simulink model "Lab_Practice_7_1simulink"  (R2024b)
settings: Solver=ode45  StartTime=0.0  StopTime=t_sim  MaxStep=0.01*Ts  MinStep=0.001*Ts  RelTol=1e-3
values from neighbouring files (symbols this model uses):
  C = [1 0]    [Es1_l7.m]    (also in Lab_Practice_7_1.m; Lab_Practice_7_1.mat; MPC_example_10_12.m = [600 0]; MPC_ratevariation.m = [600 0])
  md = MPCInit(Ad,Bd,Cy,Cz,Dz,Cc,Dc,Hp,Hw,z_blk,Hu,u_blk,du_max,du_min,u_max,u_min,z_max,z_min,Q,R,[],[],h,cmode,'qp_as')    [Es1_l7.m]    (also in Lab_Practice_7_1.m = MPCInit(Ad,Bd,Cy,Cz,Dz,Cc,Dc,Hp,Hw, z_blk, Hc, u_blk, du_max; Lab_Practice_7_1.mat = ; MPC_example_10_12.m; MPC_ratevariation.m)
  Ts = 0.05    [Es1_l7.m]    (also in Lab_Practice_7_1.m; Lab_Practice_7_1.mat; MPC_example_10_12.m = 0.001; MPC_ratevariation.m = 0.001)
  x0 = [1; 0]    [Es1_l7.m]    (also in Lab_Practice_7_1.m = [1;0]; Lab_Practice_7_1.mat = [1 0]; MPC_example_10_12.m = [0;0]; MPC_ratevariation.m = [-0.25;0])
libraries: cstblocks x1
settings Model: Creator=filoz  LastModifiedBy=filoz
settings SolverCC: InitialStep=0.001*Ts

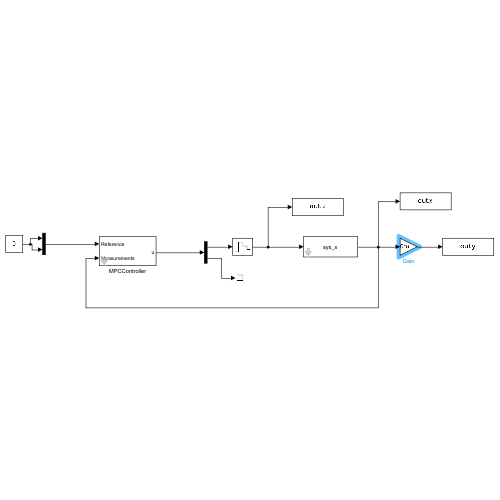
[thumbnail: Simulink's stored preview of the top-level diagram]
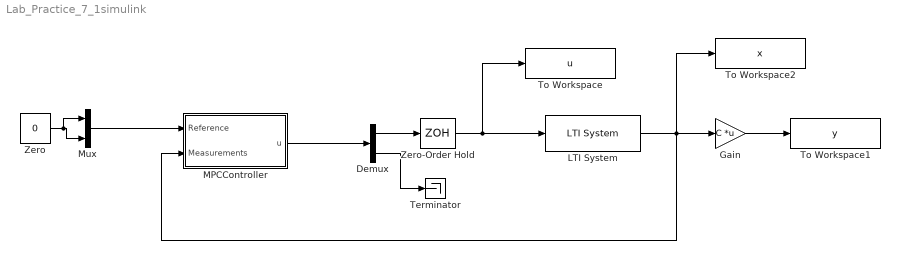
== system Lab_Practice_7_1simulink ==
  Demux : Demux  Outputs=2
  Gain : Gain  Gain=C  Multiplication=Matrix(K*u)
  LTI System : cstblocks/LTI System  sys=sys_x  IC=[x0]  PadeOrder=0
  MPCController : Subsystem  mask{md=md}
      mask prompts: md "MPCData"
  Mux : Mux  Inputs=2
  Terminator : Terminator
  To Workspace : ToWorkspace  VariableName=u  SaveFormat=Timeseries  SampleTime=0.01*Ts
  To Workspace1 : ToWorkspace  VariableName=y  SaveFormat=Timeseries  SampleTime=0.01*Ts
  To Workspace2 : ToWorkspace  VariableName=x  SaveFormat=Timeseries  SampleTime=0.01*Ts
  Zero : Constant  Value=0  OutDataTypeStr=Inherit: Inherit via back propagation
  Zero-Order Hold : ZeroOrderHold  SampleTime=Ts
  wires:
  Zero/1 -> Mux/2, Mux/1
  Mux/1 -> MPCController/1(Reference)
  MPCController/1(u) -> Demux/1
  Demux/1 -> Zero-Order Hold/1
  Zero-Order Hold/1 -> To Workspace/1, LTI System/1
  Demux/2 -> Terminator/1
  LTI System/1 -> To Workspace2/1, MPCController/2(Measurements), Gain/1
  Gain/1 -> To Workspace1/1

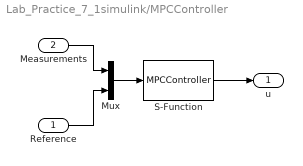
== system Lab_Practice_7_1simulink/MPCController ==
  Reference : Inport
  Measurements : Inport  Port=2
  Mux : Mux  Inputs=2
  S-Function : S-Function  FunctionName=MPCController  Parameters=md  SFunctionDeploymentMode=off  EnableBusSupport=off
  u : Outport
  wires:
  Mux/1 -> S-Function/1
  Measurements/1 -> Mux/1
  Reference/1 -> Mux/2
  S-Function/1 -> u/1
